simulink model "Matriz_CARIMA_Simulink"  (R2015a)
settings: Solver=ode45  StartTime=0.0  StopTime=20  RelTol=1e-3
values from neighbouring files (symbols this model uses):
  kgp = k*Gp    [GPCgen.m]
  kr = k*W    [GPCgen.m]
  Ts = 1    [Exercicio_1_GPC.m]
undefined symbols (not defined in the file or in its folder): kf
settings Model: Creator=Vinícius  LastModifiedBy=Vinícius

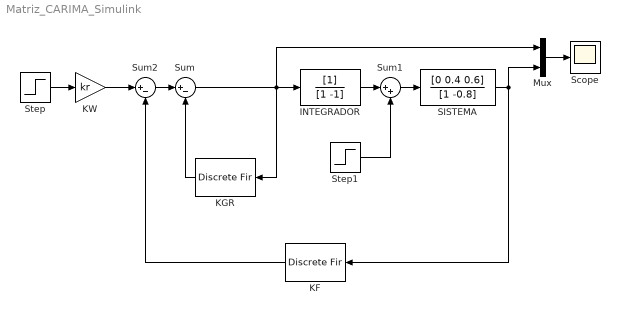
== system Matriz_CARIMA_Simulink ==
  INTEGRADOR : DiscreteFilter  Denominator=[1 -1]  SampleTime=Ts
  KF : DiscreteFir  Coefficients=kf  SampleTime=Ts
  KGR : DiscreteFir  Coefficients=[0 kgp]  SampleTime=Ts
  KW : Gain  Gain=kr
  Mux : Mux  Inputs=2
  SISTEMA : DiscreteFilter  Numerator=[0 0.4 0.6]  Denominator=[1 -0.8]  SampleTime=Ts
  Scope : Scope
  Step : Step  Time=0  SampleTime=0
  Step1 : Step  Time=10  After=-0.7  SampleTime=0
  Sum : Sum  Inputs=|+-
  Sum1 : Sum  Inputs=|++
  Sum2 : Sum  Inputs=|+-
  wires:
  SISTEMA/1 -> KF/1, Mux/2
  Step/1 -> KW/1
  Sum/1 -> KGR/1, Mux/1, INTEGRADOR/1
  KF/1 -> Sum2/2
  KGR/1 -> Sum/2
  Mux/1 -> Scope/1
  Sum2/1 -> Sum/1
  KW/1 -> Sum2/1
  INTEGRADOR/1 -> Sum1/1
  Sum1/1 -> SISTEMA/1
  Step1/1 -> Sum1/2
